simulink model "LBR_MED_CLIK"  (R2026a)
settings: Solver=ode45  StopTime=10
settings Model: Creator=ivovilamowski  LastModifiedBy=ivovilamowski

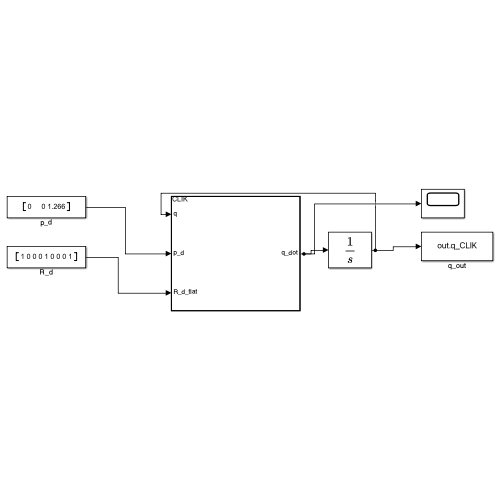
[thumbnail: Simulink's stored preview of the top-level diagram]
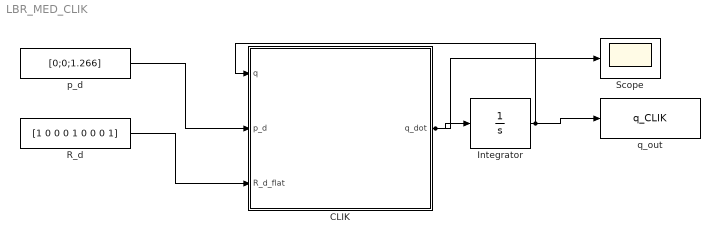
== system LBR_MED_CLIK ==
  CLIK : MATLAB Function  TreatAsAtomicUnit=on
  Integrator : Integrator  InitialCondition=[0.1;0.1;0;0.1;0;0.1;0]
  R_d : Constant  Value=[1 0 0 0 1 0 0 0 1]  OutDataTypeStr=double
  Scope : Scope
  p_d : Constant  Value=[0;0;1.266]  OutDataTypeStr=double
  q_out : ToWorkspace  VariableName=q_CLIK  SampleTime=-1
  wires:
  Integrator/1 -> CLIK/1(q), q_out/1
  p_d/1 -> CLIK/2(p_d)
  R_d/1 -> CLIK/3(R_d_flat)
  CLIK/1(q_dot) -> Integrator/1, Scope/1

== matlab function LBR_MED_CLIK/CLIK ==
  data: q input; q_dot output; p_d input; R_d_flat input
function q_dot = CLIK(q, p_d, R_d_flat)
q_dot = CLIK_law(q, p_d, R_d_flat);
end
